simulink model "multi"  (Simulink 6.0)
settings: Solver=ode1  SolverMode=SingleTasking  StartTime=0.0  StopTime=999999  MaxStep=10  RelTol=1e-3  AbsTol=1e-6
PreLoadFcn:
  | multidat
values from neighbouring files (symbols this model uses):
  a = [-1.2448    0.2015   -0.4687    0.1289    0.6421 ... (first row only)    [multidat.m]
  b = [-0.0627   -0.1878   -0.7117 ... (first row only)    [multidat.m]    (also in sfcndemo_hg_gui_m.m = get(hFig,'UserData'))
  c = [-0.6117    0.2324   -1.9889    0.5999         0 ... (first row only)    [multidat.m]
  d = [-0.1134   -2.4610   -0.7063 ... (first row only)    [multidat.m]
settings Model: Creator=The MathWorks Inc.  LastModifiedBy=batserve  ExtModeTrigMode=oneshot  ExtModeAutoUpdateStatusClock=off
settings DataIOCC: ExternalInput=[]  InitialState=[]  LimitDataPoints=off  SaveOutput=off  SaveTime=off
settings OptimizationCC: BooleanDataType=off
settings DebuggingCC: CheckExecutionContextPreStartOutputMsg=on  CheckExecutionContextRuntimeOutputMsg=on  SolverPrmCheckMsg=none
settings HardwareCC: TargetUnknown=on

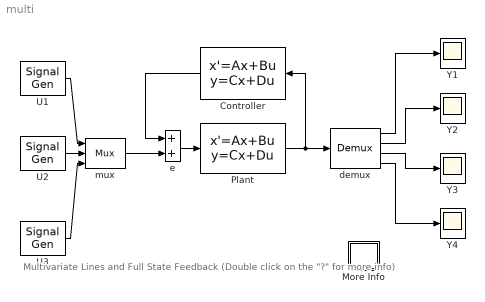
== system multi ==
  note: Multivariate Lines and  Full State Feedback
      | (Double click on the "?" for more info)
  Controller : StateSpace  Orientation=left  A=eye(size(a))  B=ones(size(c'))  C=ones(size(b'))  D=zeros(size(d'))
  More Info : Subsystem  PropExecContextAcrossSSBoundary=on
      mask Display: disp('?')
  Plant : StateSpace  A=a  B=b  C=c  D=d
  U1 : SignalGenerator  Amplitude=0.491200  Frequency=4.000000  Units=rad/sec
  U2 : SignalGenerator  Amplitude=0.130000  Frequency=6.000000  Units=rad/sec
  U3 : SignalGenerator  Amplitude=0.160000  Frequency=1.000000  Units=rad/sec
  Y{1..4} (4 alike) : Scope
      Y1 settings: TickLabels=on  TimeRange=1e+06  YMin=-3e+265  YMax=1e+265  DataFormat=Array
      Y2 settings: TickLabels=on  TimeRange=1e+06  YMin=0  YMax=2e+265  DataFormat=Array
      Y3 settings: TickLabels=on  TimeRange=1e+06  YMin=-2e+264  YMax=5e+263  DataFormat=Array
      Y4 settings: TickLabels=on  TimeRange=1e+06  YMin=-1.5e+265  YMax=5e+264  DataFormat=Array
  demux : Demux
  e : Sum  SaturateOnIntegerOverflow=on  InputSameDT=on
  mux : Mux  Inputs=3
  wires:
  demux/4 -> Y4/1
  demux/1 -> Y1/1
  demux/3 -> Y3/1
  demux/2 -> Y2/1
  Plant/1 -> demux/1, Controller/1
  Controller/1 -> e/1
  mux/1 -> e/2
  e/1 -> Plant/1
  U1/1 -> mux/1
  U2/1 -> mux/2
  U3/1 -> mux/3

== system multi/More Info ==
  note: This demonstration shows how multivariate lines can be
      | used for full state feedback and control of a MIMO system.
  note: Use the signal generators and scopes to observe how
      | the system is modeled, or try to improve the controller.
